simulink model "hign_order_fixed_time_tracking_2016"  (R2018a)
settings: Solver=ode4  StartTime=0.0  StopTime=30  FixedStep=0.001  RelTol=1e-3  EnableMultiTasking=on
settings Model: ExtModeTrigMode=oneshot  ExtModeArmWhenConnect=off  Creator=hp  LastModifiedBy=Administrator
settings DataIOCC: SaveFormat=Array  SignalLoggingSaveFormat=ModelDataLogs  SignalLoggingName=sigsOut
settings OptimizationCC: BooleanDataType=off  ExpressionDepthLimit=2147483647  InitFltsAndDblsToZero=on  LifeSpan=inf
settings DebuggingCC: SaveWithParameterizedLinksMsg=none  UnderspecifiedInitializationDetection=Classic  MergeDetectMultiDrivingBlocksExec=none  SignalResolutionControl=TryResolveAllWithWarning  MultiTaskDSMMsg=warning  MultiTaskCondExecSysMsg=none  FcnCallInpInsideContextMsg=warning  StateNameClashWarn=warning  LibraryContextMissingDiagnostic=warning  SFUnexpectedBacktrackingDiag=warning  SFNoUnconditionalDefaultTransitionDiag=warning  SFExecutionAtInitializationDiag=none
settings HardwareCC: ProdBitPerPointer=32  ProdBitPerSizeT=32  ProdBitPerPtrDiffT=32  ProdLargestAtomicFloat=None  ProdIntDivRoundTo=Undefined  ProdEndianess=Unspecified  ProdWordSize=32  ProdHWDeviceType=32-bit Generic  TargetUnknown=on
settings ModelReferenceCC: PropagateSignalLabelsOutOfModel=off
settings CodeAppCC: StateflowObjectComments=on
settings GRTTargetCC: TargetFcnLib=ansi_tfl_tmw.mat  TargetLangStandard=C89/C90 (ANSI)  GeneratePreprocessorConditionals=Disable all  CombineOutputUpdateFcns=off  GRTInterface=on
settings ConfigComp: CovMetricSettings=dw  CovHtmlReporting=on  CovSaveCumulativeToWorkspaceVar=on  CovSaveSingleToWorkspaceVar=on  CovExternalEMLEnable=off

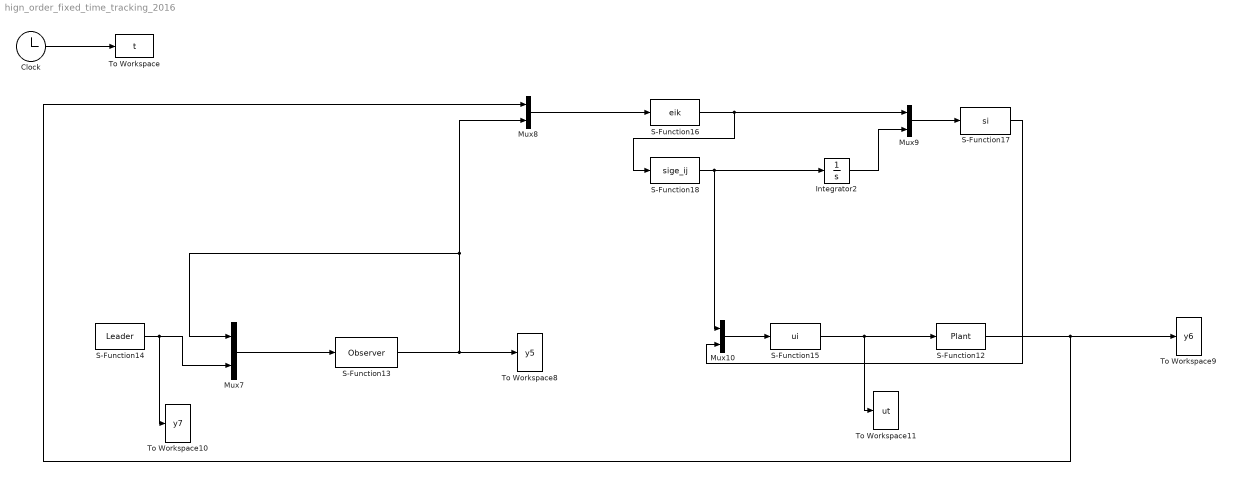
== system hign_order_fixed_time_tracking_2016 ==
  Clock : Clock
  Integrator2 : Integrator
  Mux{7..10} (4 alike) : Mux  Inputs=2
  S-Function12 : S-Function  FunctionName=Plant  SFunctionDeploymentMode=off  EnableBusSupport=off
  S-Function13 : S-Function  FunctionName=Observer  SFunctionDeploymentMode=off  EnableBusSupport=off
  S-Function14 : S-Function  FunctionName=Leader  SFunctionDeploymentMode=off  EnableBusSupport=off
  S-Function15 : S-Function  FunctionName=ui  SFunctionDeploymentMode=off  EnableBusSupport=off
  S-Function16 : S-Function  FunctionName=eik  SFunctionDeploymentMode=off  EnableBusSupport=off
  S-Function17 : S-Function  FunctionName=si  SFunctionDeploymentMode=off  EnableBusSupport=off
  S-Function18 : S-Function  FunctionName=sige_ij  SFunctionDeploymentMode=off  EnableBusSupport=off
  To Workspace : ToWorkspace  VariableName=t  SampleTime=-1
  To Workspace10 : ToWorkspace  VariableName=y7  SampleTime=-1
  To Workspace11 : ToWorkspace  VariableName=ut  SampleTime=-1
  To Workspace8 : ToWorkspace  VariableName=y5  SampleTime=-1
  To Workspace9 : ToWorkspace  VariableName=y6  SampleTime=-1
  wires:
  Clock/1 -> To Workspace/1
  S-Function12/1 -> Mux8/1, To Workspace9/1
  Mux7/1 -> S-Function13/1
  S-Function13/1 -> Mux8/2, Mux7/1, To Workspace8/1
  S-Function14/1 -> To Workspace10/1, Mux7/2
  S-Function15/1 -> To Workspace11/1, S-Function12/1
  Mux8/1 -> S-Function16/1
  S-Function16/1 -> S-Function18/1, Mux9/1
  Mux9/1 -> S-Function17/1
  S-Function18/1 -> Mux10/1, Integrator2/1
  Integrator2/1 -> Mux9/2
  Mux10/1 -> S-Function15/1
  S-Function17/1 -> Mux10/2
